simulink model "Simulink_Pendulum_Control_Offline"  (R2022b)
settings: Solver=ode1  StartTime=0.0  StopTime=10  FixedStep=0.002  RelTol=1e-3
undefined symbols (not defined in the file or in its folder): A, A_ob, alpha_max, B_ob, B_u, C_full, C_ob, D_full_u, D_ob, id_param, K_lq_alpha, Ken_eta, theta_max, voltage_max, x0
settings Model: Creator=utente  LastModifiedBy=federicocorso
settings SolverCC: AlgebraicLoopSolver=TrustRegion
settings DebuggingCC: UnconnectedInputMsg=warning  UnconnectedOutputMsg=warning  UnconnectedLineMsg=warning  SFMachineParentedDataDiag=warning
settings ModelReferenceCC: EnableRefExpFcnMdlSchedulingChecks=on

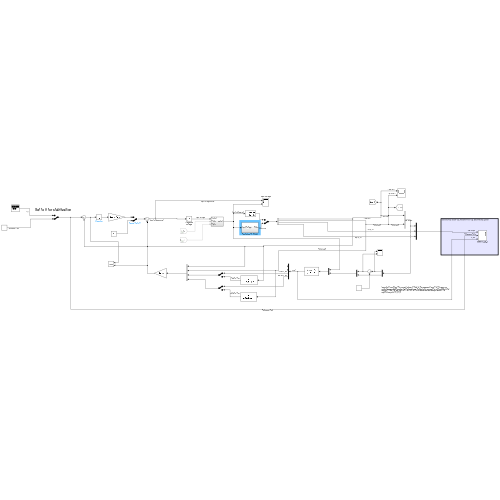
[thumbnail: Simulink's stored preview of the top-level diagram]
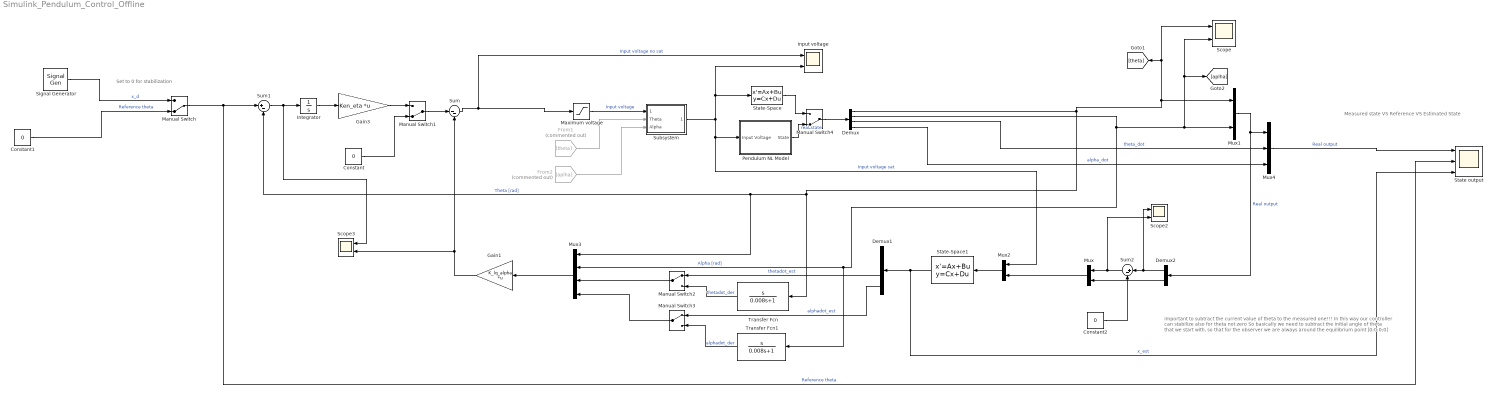
== system Simulink_Pendulum_Control_Offline ==
  note: important to subtract the current value of theta to the measured one!!! In this way our controller can stabilize also for theta not zero So basically we need to subtract the initial angle of theta that we start with, so that for the observer we are always around the equilibrium point [0;0;0;0]
  note: Measured state VS Reference VS Estimated State
  note: Set to 0 for stabilization
  Constant : Constant  Value=0
  Constant1 : Constant  Value=0
  Constant2 : Constant  Value=0
  Demux : Demux
  Demux1 : Demux
  Demux2 : Demux  Outputs=2
  From1 : From  Commented=on  GotoTag=theta
  From2 : From  Commented=on  GotoTag=aplha
  Gain1 : Gain  Gain=K_lq_alpha  Multiplication=Matrix(K*u) (u vector)
  Gain3 : Gain  Gain=Ken_eta  Multiplication=Matrix(K*u) (u vector)
  Input voltage : Scope  NumInputPorts=2
  Integrator : Integrator  LimitOutput=on  UpperSaturationLimit=3  LowerSaturationLimit=-3
  Manual Switch : ManualSwitch  CurrentSetting=0
  Manual Switch1 : ManualSwitch  CurrentSetting=0
  Manual Switch2 : ManualSwitch
  Manual Switch3 : ManualSwitch
  Manual Switch4 : ManualSwitch  CurrentSetting=0
  Maximum voltage : Saturate  UpperLimit=voltage_max  LowerLimit=-voltage_max
  Mux : Mux  Inputs=2
  Mux1 : Mux  Inputs=2
  Mux2 : Mux  Inputs=2
  Mux3 : Mux
  Mux4 : Mux  Inputs=3
  Pendulum NL Model : Subsystem
  Scope : Scope  NumInputPorts=2
  Scope2 : Scope  NumInputPorts=2
  Scope3 : Scope  NumInputPorts=2
  Signal Generator : SignalGenerator  WaveForm=square  Amplitude=0.3  Frequency=0.1
  State output : Scope  NumInputPorts=3
  State-Space : StateSpace  A=A  B=B_u  C=C_full  D=D_full_u  InitialCondition=x0
  State-Space1 : StateSpace  A=A_ob  B=B_ob  C=C_ob  D=D_ob  InitialCondition=[0;0;0;0]
  Subsystem : Subsystem
  Sum : Sum  Inputs=|--
  Sum1 : Sum  Inputs=|+-
  Sum2 : Sum  Inputs=|+-
  Transfer Fcn : TransferFcn  Numerator=[1 0]  Denominator=[0.008 1]
  Transfer Fcn1 : TransferFcn  Numerator=[1 0]  Denominator=[0.008 1]
  wires:
  Manual Switch2/1 -> Mux3/3
  Manual Switch3/1 -> Mux3/4
  Demux1/4 -> Manual Switch3/1  "alphadot_est"
  Constant/1 -> Manual Switch1/2
  Sum1/1 -> Scope3/1, Integrator/1
  Transfer Fcn/1 -> Manual Switch2/2  "thetadot_der"
  Mux3/1 -> Gain1/1
  Integrator/1 -> Gain3/1
  Gain3/1 -> Manual Switch1/1
  Demux/2 -> Mux3/2, Transfer Fcn1/1, Mux1/2, [aplha], Scope/2  "Alpha [rad]"
  Transfer Fcn1/1 -> Manual Switch3/2  "alphadot_der"
  Mux2/1 -> State-Space1/1
  Demux/1 -> Mux1/1, Scope/1, [theta], Transfer Fcn/1, Mux3/1, Sum1/2  "Theta [rad]"
  From2/1 -> Subsystem/3(Alpha)
  From1/1 -> Subsystem/2(Theta)
  Subsystem/1(control) -> Input voltage/2, State-Space/1, Pendulum NL Model/1(Input Voltage), Mux2/1  "Input voltage sat"
  Gain1/1 -> Sum/2, Scope3/2
  Manual Switch/1 -> State output/2, Sum1/1  "Reference theta"
  Mux1/1 -> Demux2/1, Mux4/1  "Real output"
  Constant1/1 -> Manual Switch/2  "Reference theta"
  Signal Generator/1 -> Manual Switch/1  "x_d"
  Sum/1 -> Maximum voltage/1, Input voltage/1  "Input voltage no sat"
  Demux1/3 -> Manual Switch2/1  "thetadot_est"
  State-Space1/1 -> Demux1/1, State output/3  "x_est"
  Maximum voltage/1 -> Subsystem/1(Control)  "Input voltage"
  Manual Switch1/1 -> Sum/1
  State-Space/1 -> Manual Switch4/1
  Demux/3 -> Mux4/2  "theta_dot"
  Demux/4 -> Mux4/3  "alpha_dot"
  Mux4/1 -> State output/1  "Real output"
  Manual Switch4/1 -> Demux/1
  Pendulum NL Model/1(State) -> Manual Switch4/2  "real state"
  Mux/1 -> Mux2/2
  Demux2/2 -> Mux/2
  Demux2/1 -> Scope2/1, Sum2/1
  Sum2/1 -> Scope2/2, Mux/1
  Constant2/1 -> Sum2/2

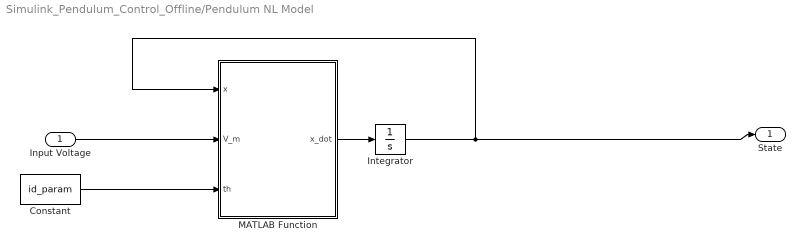
== system Simulink_Pendulum_Control_Offline/Pendulum NL Model ==
  Input Voltage : Inport
  Constant : Constant  Value=id_param
  Integrator : Integrator  InitialCondition=x0
  MATLAB Function : MATLAB Function  TreatAsAtomicUnit=on
  State : Outport
  wires:
  Input Voltage/1 -> MATLAB Function/2(V_m)
  Constant/1 -> MATLAB Function/3(th)
  MATLAB Function/1(x_dot) -> Integrator/1
  Integrator/1 -> MATLAB Function/1(x), State/1

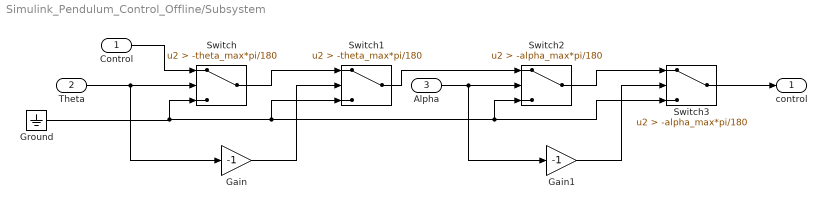
== system Simulink_Pendulum_Control_Offline/Subsystem ==
  Control : Inport
  Theta : Inport  Port=2
  Alpha : Inport  Port=3
  Gain : Gain  Gain=-1
  Gain1 : Gain  Gain=-1
  Ground : Ground
  Switch : Switch  Criteria=u2 > Threshold  Threshold=-theta_max*pi/180  SaturateOnIntegerOverflow=off  InputSameDT=off
  Switch1 : Switch  Criteria=u2 > Threshold  Threshold=-theta_max*pi/180  SaturateOnIntegerOverflow=off  InputSameDT=off
  Switch2 : Switch  Criteria=u2 > Threshold  Threshold=-alpha_max*pi/180  SaturateOnIntegerOverflow=off  InputSameDT=off
  Switch3 : Switch  Criteria=u2 > Threshold  Threshold=-alpha_max*pi/180  SaturateOnIntegerOverflow=off  InputSameDT=off
  control : Outport
  wires:
  Gain/1 -> Switch1/2
  Theta/1 -> Gain/1, Switch/2
  Control/1 -> Switch/1
  Switch/1 -> Switch1/1
  Gain1/1 -> Switch3/2
  Switch1/1 -> Switch2/1
  Ground/1 -> Switch3/3, Switch2/3, Switch1/3, Switch/3
  Switch2/1 -> Switch3/1
  Alpha/1 -> Switch2/2, Gain1/1
  Switch3/1 -> control/1

== matlab function Simulink_Pendulum_Control_Offline/Pendulum NL Model/MATLAB Function ==
  data: x input; x_dot output; V_m input; th input
function x_dot = NL_eqns(x,V_m,th)
%NL_eqns
%    NL_DIFF_EQNS_SS = NL_eqns(B_p,B_r,J_a,J_p,G,L_P,M_P,R,TAU,x(2,1),x(3,1),x(4,1),X_DOT_1,X_DOT_2,X_DOT_3,X_DOT_4)

%    This function was generated by the Symbolic Math Toolbox version 9.2.
%    09-Mar-2023 15:34:15
B_p = th(1,1);
B_r = th(2,1);
J_a = th(3,1);
J_p = th(4,1);
l_p = th(5,1);
m_p = th(6,1);
r = th(7,1);
g = th(8,1);
K_g = th(9,1);
R_m = th(10,1);
eta_g = th(11,1);
eta_m = th(12,1);
k_m = th(13,1);
k_t = th(14,1);

tau = eta_g*K_g*eta_m*k_t*(V_m-K_g*k_m*x(3,1))/R_m; % motor torque expression-STATIC

t2 = cos(x(2,1));
t3 = sin(x(2,1));
t4 = l_p.^2;
t5 = l_p.^3;
t7 = m_p.^2;
t8 = r.^2;
t9 = x(2,1).*2.0;
t10 = x(3,1).^2;
t11 = x(4,1).^2;
t12 = J_a.*J_p;
t6 = t4.^2;
t13 = t2.^2;
t14 = sin(t9);
t15 = J_a.*m_p.*t4;
t16 = J_p.*m_p.*t4;
t17 = J_p.*m_p.*t8;
t20 = t4.*t7.*t8;
t18 = t6.*t7;
t19 = t13.*t16;
t24 = t13.*t20;
t21 = t13.*t18;
t22 = -t19;
t25 = -t24;
t23 = -t21;
t26 = t12+t15+t16+t17+t18+t20+t22+t23+t25;
t27 = 1.0./t26;

x_dot = zeros(4,1);

x_dot(1,1) = x(3,1);
x_dot(2,1) = x(4,1);
x_dot(3,1) = t27.*(J_p.*tau.*-2.0+B_r.*J_p.*x(3,1).*2.0-m_p.*t4.*tau.*2.0+t14.*t16.*x(3,1).*x(4,1).*2.0+t14.*t18.*x(3,1).*x(4,1).*2.0+B_r.*m_p.*t4.*x(3,1).*2.0+r.*t3.*t5.*t7.*t11.*2.0-g.*r.*t2.*t3.*t4.*t7.*2.0-r.*t2.*t5.*t7.*t10.*t14+B_p.*l_p.*m_p.*r.*t2.*x(4,1).*2.0+J_p.*l_p.*m_p.*r.*t3.*t11.*2.0).*(-1.0./2.0);
x_dot(4,1) = t27.*(B_p.*J_a.*x(4,1).*2.0-t10.*t14.*t15-t10.*t14.*t18-t10.*t14.*t20+t10.*t14.*t21-g.*t3.*t5.*t7.*2.0+t2.*t3.*t11.*t20.*2.0+B_p.*m_p.*t4.*x(4,1).*2.0+B_p.*m_p.*t8.*x(4,1).*2.0-J_a.*g.*l_p.*m_p.*t3.*2.0-B_p.*m_p.*t4.*t13.*x(4,1).*2.0-g.*l_p.*t3.*t7.*t8.*2.0-l_p.*m_p.*r.*t2.*tau.*2.0+g.*t3.*t5.*t7.*t13.*2.0+B_r.*l_p.*m_p.*r.*t2.*x(3,1).*2.0+r.*t2.*t5.*t7.*t14.*x(3,1).*x(4,1).*2.0).*(-1.0./2.0);

% x_plus_1 = zeros(4,1);
% x_plus_1 = x + Ts*x_dot;

% x_plus_1(1,1) = x(1,1) + Ts*x_dot(1,1);
% x_plus_1(1,1) = x(1,1) + Ts*x_dot(1,1);
% x_plus_1(1,1) = x(1,1) + Ts*x_dot(1,1);
% x_plus_1(1,1) = x(1,1) + Ts*x_dot(1,1);
